simulink model "stage_manager_test"  (R2024b)
settings: Solver=FixedStepDiscrete  StartTime=0.0  StopTime=2  FixedStep=0.05  RelTol=1e-3
libraries: simulink x3
settings Model: Creator=aiden  LastModifiedBy=aiden

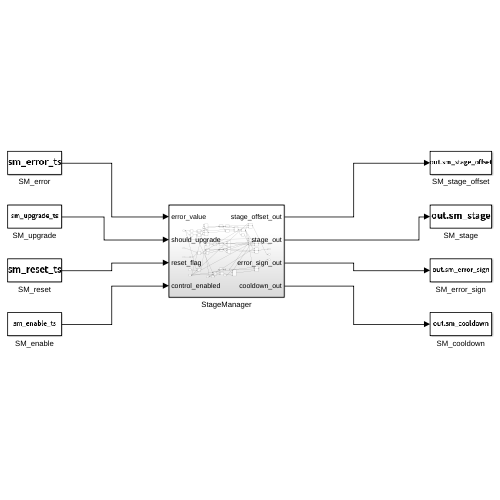
[thumbnail: Simulink's stored preview of the top-level diagram]
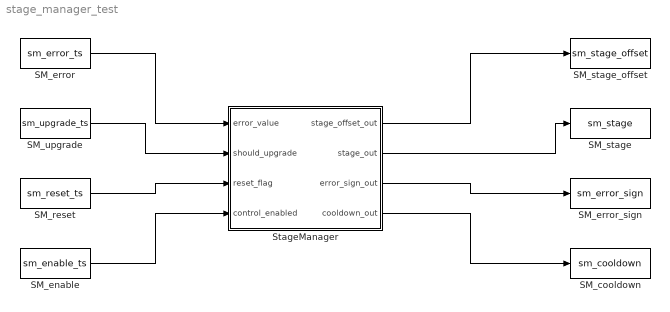
== system stage_manager_test ==
  SM_cooldown : ToWorkspace  VariableName=sm_cooldown  SaveFormat=Structure With Time  SampleTime=-1
  SM_enable : FromWorkspace  VariableName=sm_enable_ts
  SM_error : FromWorkspace  VariableName=sm_error_ts
  SM_error_sign : ToWorkspace  VariableName=sm_error_sign  SaveFormat=Structure With Time  SampleTime=-1
  SM_reset : FromWorkspace  VariableName=sm_reset_ts
  SM_stage : ToWorkspace  VariableName=sm_stage  SaveFormat=Structure With Time  SampleTime=-1
  SM_stage_offset : ToWorkspace  VariableName=sm_stage_offset  SaveFormat=Structure With Time  SampleTime=-1
  SM_upgrade : FromWorkspace  VariableName=sm_upgrade_ts
  StageManager : Subsystem
  wires:
  SM_error/1 -> StageManager/1(error_value)
  SM_upgrade/1 -> StageManager/2(should_upgrade)
  SM_reset/1 -> StageManager/3(reset_flag)
  SM_enable/1 -> StageManager/4(control_enabled)
  StageManager/1(stage_offset_out) -> SM_stage_offset/1
  StageManager/2(stage_out) -> SM_stage/1
  StageManager/3(error_sign_out) -> SM_error_sign/1
  StageManager/4(cooldown_out) -> SM_cooldown/1

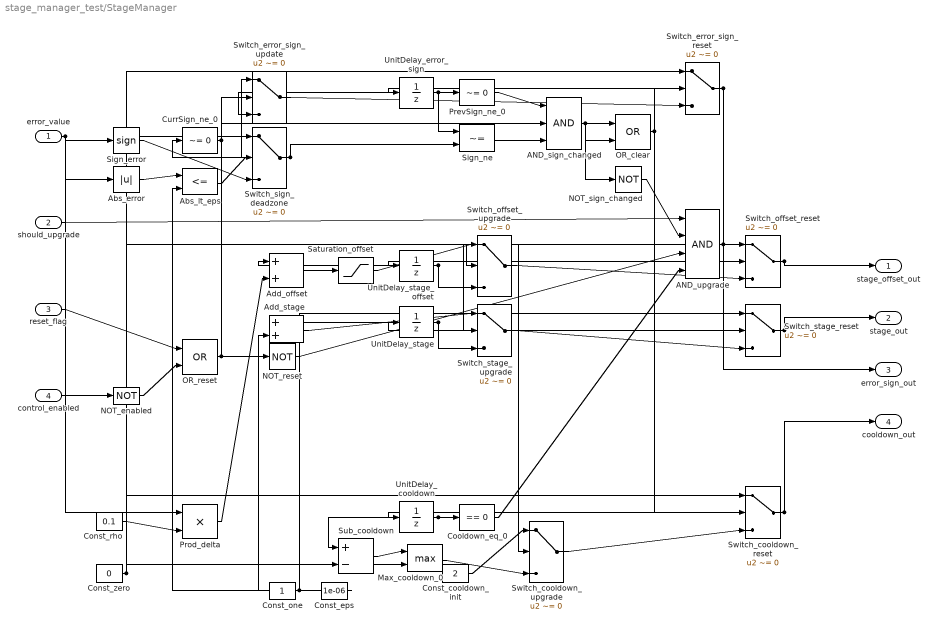
== system stage_manager_test/StageManager ==
  error_value : Inport
  should_upgrade : Inport  Port=2
  reset_flag : Inport  Port=3
  control_enabled : Inport  Port=4
  AND_sign_changed : Logic  Inputs=3  AllPortsSameDT=off  OutDataTypeStr=boolean
  AND_upgrade : Logic  Inputs=4  AllPortsSameDT=off  OutDataTypeStr=boolean
  Abs_error : Abs  SaturateOnIntegerOverflow=off
  Abs_lt_eps : RelationalOperator  Operator=<=  OutDataTypeStr=boolean  RndMeth=Simplest  InputSameDT=off
  Add_offset : Sum
  Add_stage : Sum
  Const_cooldown_init : Constant  Value=2
  Const_eps : Constant  Value=1e-06
  Const_one : Constant
  Const_rho : Constant  Value=0.1
  Const_zero : Constant  Value=0
  Cooldown_eq_0 : simulink/Logic and Bit Operations/Compare To Zero  relop===  OutDataTypeStr=boolean
  CurrSign_ne_0 : simulink/Logic and Bit Operations/Compare To Zero  relop=~=  OutDataTypeStr=boolean
  Max_cooldown_0 : MinMax  Function=max  Inputs=2
  NOT_enabled : Logic  Operator=NOT  AllPortsSameDT=off  OutDataTypeStr=boolean
  NOT_reset : Logic  Operator=NOT  AllPortsSameDT=off  OutDataTypeStr=boolean
  NOT_sign_changed : Logic  Operator=NOT  AllPortsSameDT=off  OutDataTypeStr=boolean
  OR_clear : Logic  Operator=OR  AllPortsSameDT=off  OutDataTypeStr=boolean
  OR_reset : Logic  Operator=OR  AllPortsSameDT=off  OutDataTypeStr=boolean
  PrevSign_ne_0 : simulink/Logic and Bit Operations/Compare To Zero  relop=~=  OutDataTypeStr=boolean
  Prod_delta : Product
  Saturation_offset : Saturate  UpperLimit=500  LowerLimit=-500
  Sign_error : Signum
  Sign_ne : RelationalOperator  Operator=~=  OutDataTypeStr=boolean  RndMeth=Simplest  InputSameDT=off
  Sub_cooldown : Sum  Inputs=+-
  Switch_cooldown_reset : Switch  Criteria=u2 ~= 0  SaturateOnIntegerOverflow=off  InputSameDT=off
  Switch_cooldown_upgrade : Switch  Criteria=u2 ~= 0  SaturateOnIntegerOverflow=off  InputSameDT=off
  Switch_error_sign_reset : Switch  Criteria=u2 ~= 0  SaturateOnIntegerOverflow=off  InputSameDT=off
  Switch_error_sign_update : Switch  Criteria=u2 ~= 0  SaturateOnIntegerOverflow=off  InputSameDT=off
  Switch_offset_reset : Switch  Criteria=u2 ~= 0  SaturateOnIntegerOverflow=off  InputSameDT=off
  Switch_offset_upgrade : Switch  Criteria=u2 ~= 0  SaturateOnIntegerOverflow=off  InputSameDT=off
  Switch_sign_deadzone : Switch  Criteria=u2 ~= 0  SaturateOnIntegerOverflow=off  InputSameDT=off
  Switch_stage_reset : Switch  Criteria=u2 ~= 0  SaturateOnIntegerOverflow=off  InputSameDT=off
  Switch_stage_upgrade : Switch  Criteria=u2 ~= 0  SaturateOnIntegerOverflow=off  InputSameDT=off
  UnitDelay_cooldown : UnitDelay  SampleTime=-1  HasFrameUpgradeWarning=on
  UnitDelay_error_sign : UnitDelay  SampleTime=-1  HasFrameUpgradeWarning=on
  UnitDelay_stage : UnitDelay  InitialCondition=1  SampleTime=-1  HasFrameUpgradeWarning=on
  UnitDelay_stage_offset : UnitDelay  SampleTime=-1  HasFrameUpgradeWarning=on
  stage_offset_out : Outport
  stage_out : Outport  Port=2
  error_sign_out : Outport  Port=3
  cooldown_out : Outport  Port=4
  wires:
  control_enabled/1 -> NOT_enabled/1
  reset_flag/1 -> OR_reset/1
  NOT_enabled/1 -> OR_reset/2
  error_value/1 -> Sign_error/1, Abs_error/1, Prod_delta/1
  Abs_error/1 -> Abs_lt_eps/1
  Const_eps/1 -> Abs_lt_eps/2
  Const_zero/1 -> Switch_sign_deadzone/1, Switch_offset_reset/1, Switch_error_sign_reset/1, Max_cooldown_0/2, Switch_cooldown_reset/1
  Abs_lt_eps/1 -> Switch_sign_deadzone/2
  Sign_error/1 -> Switch_sign_deadzone/3
  Switch_sign_deadzone/1 -> CurrSign_ne_0/1, Sign_ne/2, Switch_error_sign_update/1
  UnitDelay_error_sign/1 -> PrevSign_ne_0/1, Sign_ne/1, Switch_error_sign_update/3
  PrevSign_ne_0/1 -> AND_sign_changed/1
  CurrSign_ne_0/1 -> AND_sign_changed/2, Switch_error_sign_update/2
  Sign_ne/1 -> AND_sign_changed/3
  OR_reset/1 -> OR_clear/1, NOT_reset/1
  AND_sign_changed/1 -> OR_clear/2, NOT_sign_changed/1
  should_upgrade/1 -> AND_upgrade/1
  NOT_sign_changed/1 -> AND_upgrade/2
  NOT_reset/1 -> AND_upgrade/3
  UnitDelay_cooldown/1 -> Cooldown_eq_0/1, Sub_cooldown/1
  Cooldown_eq_0/1 -> AND_upgrade/4
  Const_rho/1 -> Prod_delta/2
  UnitDelay_stage_offset/1 -> Add_offset/1, Switch_offset_upgrade/3
  Prod_delta/1 -> Add_offset/2
  Add_offset/1 -> Saturation_offset/1
  Saturation_offset/1 -> Switch_offset_upgrade/1
  AND_upgrade/1 -> Switch_offset_upgrade/2, Switch_cooldown_upgrade/2, Switch_stage_upgrade/2
  OR_clear/1 -> Switch_offset_reset/2, Switch_error_sign_reset/2, Switch_cooldown_reset/2, Switch_stage_reset/2
  Switch_offset_upgrade/1 -> Switch_offset_reset/3
  Switch_offset_reset/1 -> UnitDelay_stage_offset/1, stage_offset_out/1
  Switch_error_sign_update/1 -> Switch_error_sign_reset/3
  Switch_error_sign_reset/1 -> UnitDelay_error_sign/1, error_sign_out/1
  Const_one/1 -> Sub_cooldown/2, Add_stage/2, Switch_stage_reset/1
  Sub_cooldown/1 -> Max_cooldown_0/1
  Const_cooldown_init/1 -> Switch_cooldown_upgrade/1
  Max_cooldown_0/1 -> Switch_cooldown_upgrade/3
  Switch_cooldown_upgrade/1 -> Switch_cooldown_reset/3
  Switch_cooldown_reset/1 -> UnitDelay_cooldown/1, cooldown_out/1
  UnitDelay_stage/1 -> Add_stage/1, Switch_stage_upgrade/3
  Add_stage/1 -> Switch_stage_upgrade/1
  Switch_stage_upgrade/1 -> Switch_stage_reset/3
  Switch_stage_reset/1 -> UnitDelay_stage/1, stage_out/1
